simulink model "Bias"  (R2017b)
settings: Solver=FixedStepAuto  StartTime=0.0  StopTime=10.0  FixedStep=0.200000  RelTol=1e-3  EnableMultiTasking=on
settings Model: Creator=ktrinh  LastModifiedBy=hbourbou
settings OptimizationCC: LifeSpan=inf
settings DebuggingCC: SFUnexpectedBacktrackingDiag=warning  SFNoUnconditionalDefaultTransitionDiag=warning  SFExecutionAtInitializationDiag=none
settings HardwareCC: ProdBitPerSizeT=32  ProdBitPerPtrDiffT=32  ProdWordSize=32  ProdHWDeviceType=Specified
settings CodeAppCC: StateflowObjectComments=on
settings GRTTargetCC: TargetLangStandard=C89/C90 (ANSI)  GeneratePreprocessorConditionals=Disable all
settings ConfigComp: CovMetricSettings=dw  CovHtmlReporting=on  CovSaveCumulativeToWorkspaceVar=on  CovSaveSingleToWorkspaceVar=on  CovExternalEMLEnable=off

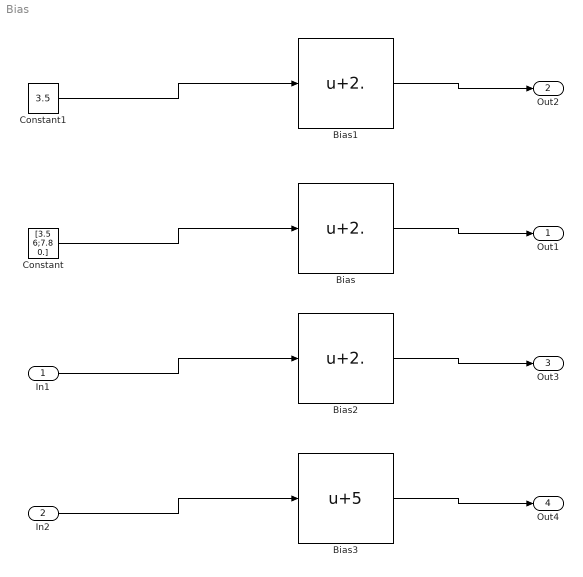
== system Bias ==
  In1 : Inport  OutDataTypeStr=double
  In2 : Inport  Port=2  OutDataTypeStr=int32
  Bias : Bias  Bias=2.  SaturateOnIntegerOverflow=on
  Bias1 : Bias  Bias=2.  SaturateOnIntegerOverflow=on
  Bias2 : Bias  Bias=2.  SaturateOnIntegerOverflow=on
  Bias3 : Bias  Bias=5  SaturateOnIntegerOverflow=on
  Constant : Constant  Value=[3.5 6;7.8 0.]
  Constant1 : Constant  Value=3.5
  Out1 : Outport
  Out2 : Outport  Port=2
  Out3 : Outport  Port=3
  Out4 : Outport  Port=4
  wires:
  Constant/1 -> Bias/1
  Bias/1 -> Out1/1
  Constant1/1 -> Bias1/1
  Bias1/1 -> Out2/1
  In1/1 -> Bias2/1
  Bias2/1 -> Out3/1
  In2/1 -> Bias3/1
  Bias3/1 -> Out4/1
